simulink model "Model02_ParaEstimation"  (R2021b)
settings: Solver=FixedStepAuto  StartTime=0.0  StopTime=T  FixedStep=Ts  RelTol=1e-3
values from neighbouring files (symbols this model uses):
  Ad = Ac*Ts+eye(2)    [KalmanFilter.m]    (also in ParaEstimation.m = Ac*Ts+eye(3); Sim01_KalmanFilter.m; Sim02_DisturbEst.m = Ac*Ts+eye(4); Sim02_ParaEstimation.m = Ac*Ts+eye(3))
  Bd = Bc*Ts    [KalmanFilter.m]    (also in ParaEstimation.m; Sim01_KalmanFilter.m; Sim02_DisturbEst.m; Sim02_ParaEstimation.m)
  Cd = Cc    [KalmanFilter.m]    (also in ParaEstimation.m; Sim01_KalmanFilter.m; Sim02_DisturbEst.m; Sim02_ParaEstimation.m)
  Fn = 1e-3    (= 0.001)    [ParaEstimation.m]    (also in Sim02_DisturbEst.m; Sim02_ParaEstimation.m)
  k = 2    [ParaEstimation.m]    (also in Sim02_DisturbEst.m; Sim02_ParaEstimation.m)
  Q = 1e-3    (= 0.001)    [KalmanFilter.m]    (also in ParaEstimation.m = diag([0 0 Fn]); Sim01_KalmanFilter.m; Sim02_DisturbEst.m = diag([0 0 Fn 0]); Sim02_ParaEstimation.m = diag([0 0 Fn]))
  R = 1e-3    (= 0.001)    [KalmanFilter.m]    (also in ParaEstimation.m; Sim01_KalmanFilter.m; Sim02_DisturbEst.m; Sim02_ParaEstimation.m)
  Ts = 1e-3    (= 0.001)    [KalmanFilter.m]    (also in ParaEstimation.m; Sim01_KalmanFilter.m; Sim02_DisturbEst.m; Sim02_ParaEstimation.m)
  x0 = 1    [ParaEstimation.m]    (also in Sim02_DisturbEst.m; Sim02_ParaEstimation.m; Sim03_ExtendedKF.m = [1 0]')
  xk = [0.8 0 0]    [ParaEstimation.m]    (also in Sim02_DisturbEst.m = [0.8 0 0 0]; Sim02_ParaEstimation.m)
libraries: simulink x2
settings Model: Creator=XiaoCY  LastModifiedBy=xiaocy
settings SolverCC: AlgebraicLoopSolver=TrustRegion
settings DataIOCC: ReturnWorkspaceOutputs=off
settings DebuggingCC: SFMachineParentedDataDiag=warning

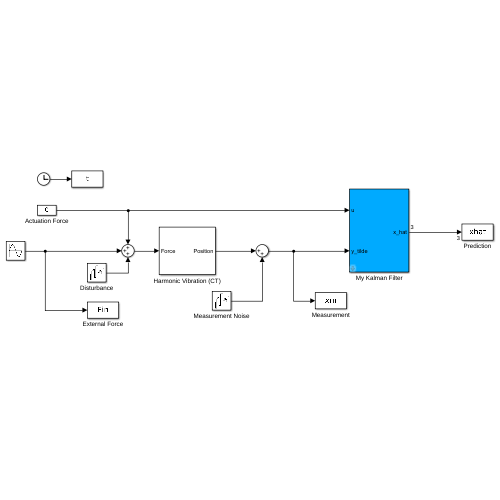
[thumbnail: Simulink's stored preview of the top-level diagram]
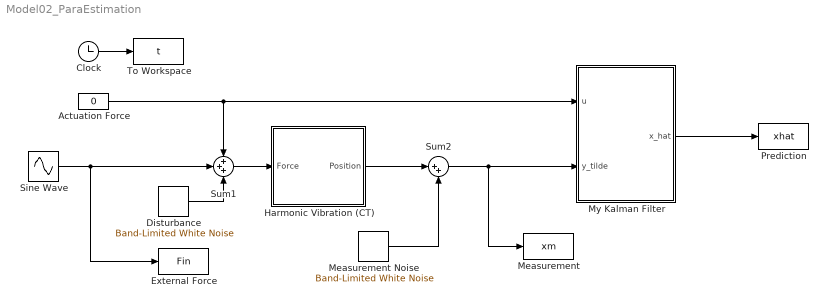
== system Model02_ParaEstimation ==
  Actuation Force : Constant  Value=0
  Clock : Clock
  Disturbance : simulink/Sources/Band-Limited White Noise  Cov=Fn*Ts  Ts=Ts  seed=[23341]
  External Force : ToWorkspace  VariableName=Fin  SampleTime=Ts
  Harmonic Vibration (CT) : Subsystem
  Measurement : ToWorkspace  VariableName=xm  SampleTime=Ts
  Measurement Noise : simulink/Sources/Band-Limited White Noise  Cov=R*Ts  Ts=Ts  seed=13412
  My Kalman Filter : Subsystem  mask{A=Ad, B=Bd, C=Cd, Q=Q, R=R, x0=xk, Ts=Ts}
      mask prompts: x0 "Initial state"
  Prediction : ToWorkspace  VariableName=xhat  SampleTime=Ts
  Sine Wave : Sin  SampleTime=0
  Sum1 : Sum  Inputs=+++
  Sum2 : Sum  Inputs=|++
  To Workspace : ToWorkspace  VariableName=t  SampleTime=Ts
  wires:
  Measurement Noise/1 -> Sum2/2
  Disturbance/1 -> Sum1/3
  My Kalman Filter/1(x_hat) -> Prediction/1
  Harmonic Vibration (CT)/1(Position) -> Sum2/1
  Sum2/1 -> My Kalman Filter/2(y_tilde), Measurement/1
  Actuation Force/1 -> My Kalman Filter/1(u), Sum1/1
  Clock/1 -> To Workspace/1
  Sum1/1 -> Harmonic Vibration (CT)/1(Force)
  Sine Wave/1 -> Sum1/2, External Force/1

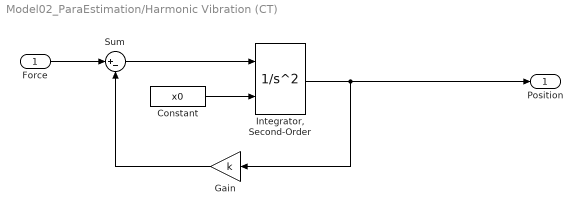
== system Model02_ParaEstimation/Harmonic Vibration (CT) ==
  Force : Inport
  Constant : Constant  Value=x0
  Gain : Gain  Gain=k
  "Integrator, Second-Order" : SecondOrderIntegrator  ICSourceX=external  ShowOutput=x
  Sum : Sum  Inputs=|+-
  Position : Outport
  wires:
  Sum/1 -> "Integrator, Second-Order"/1
  Constant/1 -> "Integrator, Second-Order"/2
  "Integrator, Second-Order"/1 -> Gain/1, Position/1
  Gain/1 -> Sum/2
  Force/1 -> Sum/1

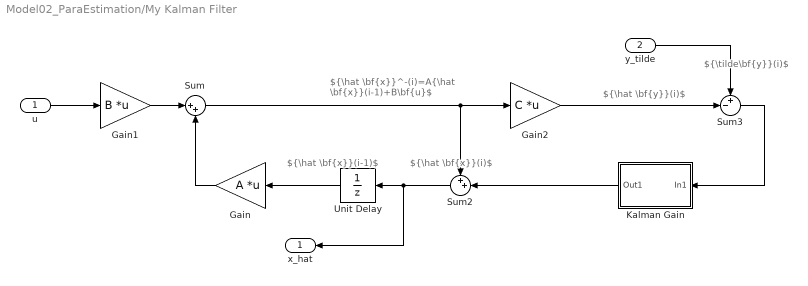
== system Model02_ParaEstimation/My Kalman Filter ==
  note: ${\hat \bf{x}}(i)$
  note: ${\hat \bf{x}}(i-1)$
  note: ${\hat \bf{x}}^-(i)=A{\hat \bf{x}}(i-1)+B\bf{u}$
  note: ${\hat \bf{y}}(i)$
  note: ${\tilde\bf{y}}(i)$
  u : Inport
  y_tilde : Inport  Port=2
  Gain : Gain  Gain=A  Multiplication=Matrix(K*u)
  Gain1 : Gain  Gain=B  Multiplication=Matrix(K*u)
  Gain2 : Gain  Gain=C  Multiplication=Matrix(K*u)
  Kalman Gain : Subsystem
      mask Display: disp('K')
  Sum : Sum  Inputs=|++
  Sum2 : Sum  Inputs=++|
  Sum3 : Sum  Inputs=+-|
  Unit Delay : UnitDelay  InitialCondition=x0  SampleTime=-1  HasFrameUpgradeWarning=on
  x_hat : Outport
  wires:
  Unit Delay/1 -> Gain/1
  Gain/1 -> Sum/2
  Gain1/1 -> Sum/1
  Sum/1 -> Gain2/1, Sum2/1
  Sum2/1 -> x_hat/1, Unit Delay/1
  Gain2/1 -> Sum3/2
  Sum3/1 -> Kalman Gain/1(In1)
  u/1 -> Gain1/1
  y_tilde/1 -> Sum3/1
  Kalman Gain/1(Out1) -> Sum2/2

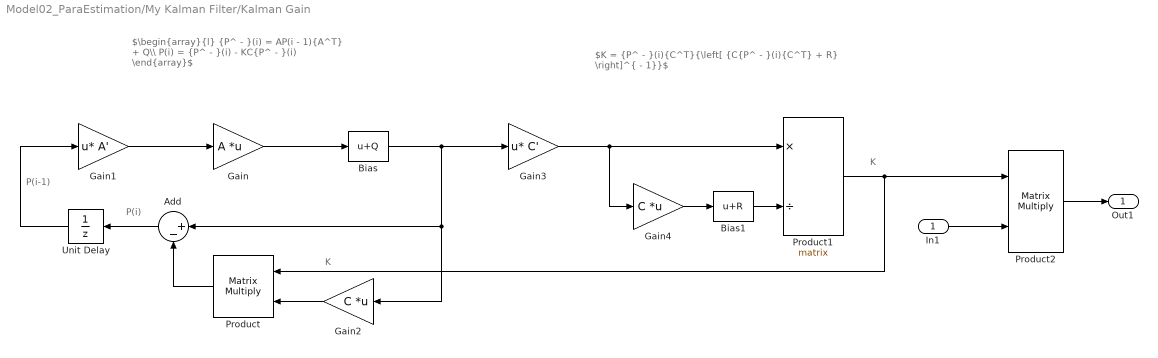
== system Model02_ParaEstimation/My Kalman Filter/Kalman Gain ==
  note: P(i)
  note: $\begin{array}{l} {P^ - }(i) = AP(i - 1){A^T} + Q\\ P(i) = {P^ - }(i) - KC{P^ - }(i) \end{array}$
  note: $K = {P^ - }(i){C^T}{\left[ {C{P^ - }(i){C^T} + R} \right]^{ - 1}}$
  note: P(i-1)
  note: K
  note: K
  In1 : Inport
  Add : Sum  Inputs=|+-
  Bias : Bias  Bias=Q
  Bias1 : Bias  Bias=R
  Gain : Gain  Gain=A  Multiplication=Matrix(K*u)
  Gain1 : Gain  Gain=A'  Multiplication=Matrix(u*K)
  Gain2 : Gain  Gain=C  Multiplication=Matrix(K*u)
  Gain3 : Gain  Gain=C'  Multiplication=Matrix(u*K)
  Gain4 : Gain  Gain=C  Multiplication=Matrix(K*u)
  Product : Product  Multiplication=Matrix(*)
  Product1 : Product  Inputs=*/  Multiplication=Matrix(*)
  Product2 : Product  Multiplication=Matrix(*)
  Unit Delay : UnitDelay  SampleTime=-1  HasFrameUpgradeWarning=on
  Out1 : Outport
  wires:
  Unit Delay/1 -> Gain1/1
  Gain1/1 -> Gain/1
  Gain/1 -> Bias/1
  Bias/1 -> Gain3/1, Gain2/1, Add/1
  Gain2/1 -> Product/2
  Product/1 -> Add/2
  Add/1 -> Unit Delay/1
  Gain3/1 -> Gain4/1, Product1/1
  Gain4/1 -> Bias1/1
  Bias1/1 -> Product1/2
  Product1/1 -> Product2/1, Product/1
  In1/1 -> Product2/2
  Product2/1 -> Out1/1
